simulink model "spacecraft2"  (R2022b)
settings: Solver=ode45  StartTime=0.0  StopTime=tf  RelTol=1e-12  AbsTol=1e-12
values from neighbouring files (symbols this model uses):
  acc = 0.5*pi/180    (= 0.00872664625997)    [runsimulink.m]
  angle0 = [0 0 0]'    [runsimulink.m]
  Jb_cg = diag([90 70 60])    [main.m]    (also in runsimulink.m)
  x0 = [rvi_0;qb_i0;wb_bi0]'    [runsimulink.m]
settings Model: Creator=fg7823  LastModifiedBy=dopestmmac
settings DebuggingCC: UnconnectedInputMsg=warning  UnconnectedOutputMsg=warning  UnconnectedLineMsg=warning
settings ModelReferenceCC: EnableRefExpFcnMdlSchedulingChecks=on
settings RTWCC: DLArmComputeVersion=19.05

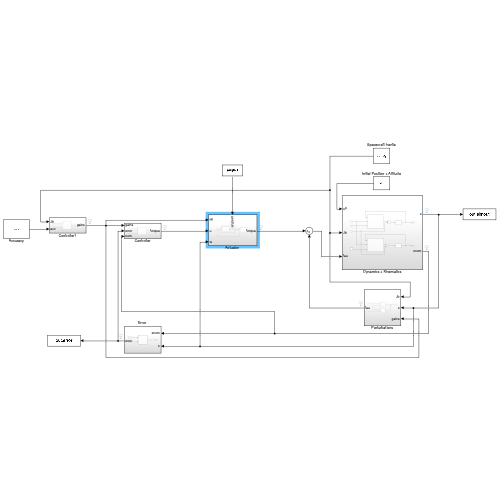
[thumbnail: Simulink's stored preview of the top-level diagram]
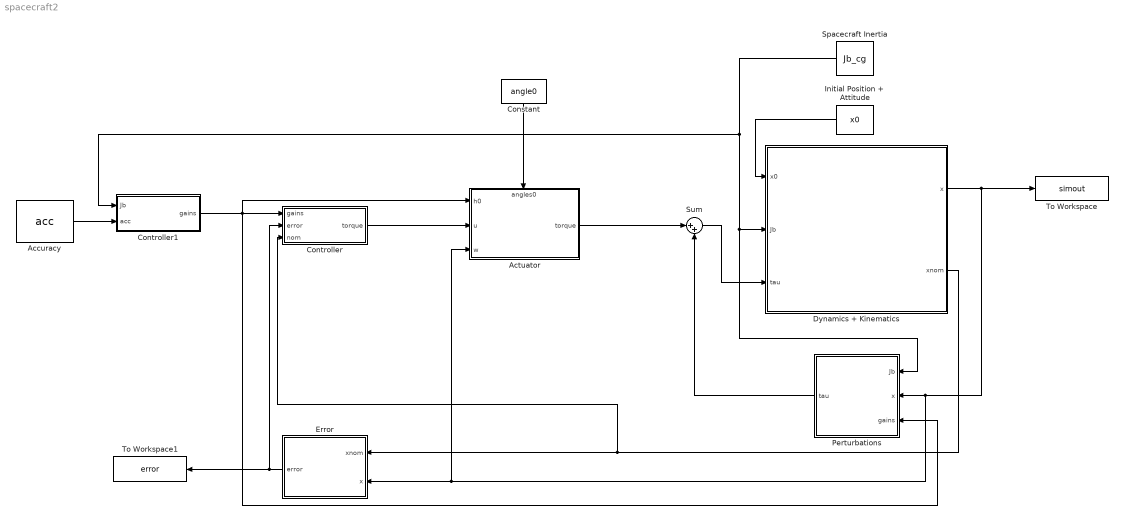
== system spacecraft2 ==
  Accuracy : Constant  Value=acc
  "Actuator " : Subsystem
      settings: PortSchema="{\"entries\":[{\"content\":{\"sides\":[{\"content\":{\"connectorIds\":[\"In1\",\"In2\",\"In3\"]},\"type\":\"ConnectorPlacement.EquallySpacedRectSide\",\"uuid\":\"5f27c84e-cce5-4eac-9877-9210f497f153\"},{\"content\":{\"connectorIds\":[\"Out1\"],\"side\":\"RIGHT\"},\"type\":\"ConnectorPlacement.EquallySpacedRectSide\",\"uuid\":\"a466bbdb-492f-41de-a900-9cb886f81e3e\"},{\"content\":{\"connectorIds\":[\"In4\"],\"side\":\"TOP\"},\"type\":\"ConnectorPlacement.EquallySpacedRectSide\",\"uuid\":\"03fb3c46-a5e4-4bdc-953c-ec3813d7b557\"},{\"content\":{\"connectorIds\":[],\"side\":\"BOTTOM\"},\"type\":\"ConnectorPlacement.EquallySpacedRectSide\",\"uuid\":\"bd57d3c1-5596-4982-b272-865ebb4241ce\"}]},\"type\":\"ConnectorPlacement.EquallySpacedConnector\",\"uuid\":\"40601c32-580e-43fd-8255-02ff6b55ccd6\"}],\"packageUris\":[\"http://schema.mathworks.com/mf0/Connector/R2020b\"],\"version\":\"1.0\"}"
  Constant : Constant  Value=angle0
  Controller : Subsystem
  Controller1 : Subsystem
  Dynamics + Kinematics : Subsystem
  "Error " : Subsystem
  Initial Position + Attitude : Constant  Value=x0
  Perturbations : Subsystem
  Spacecraft Inertia : Constant  Value=Jb_cg
  Sum : Sum  Inputs=|++
  To Workspace : ToWorkspace  VariableName=simout  SampleTime=-1
  To Workspace1 : ToWorkspace  VariableName=error  SampleTime=-1
  wires:
  Spacecraft Inertia/1 -> Controller1/1(Jb), Dynamics + Kinematics/2(Jb), Perturbations/1(Jb)
  Initial Position + Attitude/1 -> Dynamics + Kinematics/1(x0)
  Dynamics + Kinematics/1(x) -> To Workspace/1, Perturbations/2(x), "Actuator "/3(w), "Error "/2(x)
  Dynamics + Kinematics/2(xnom) -> Controller/3(nom), "Error "/1(xnom)
  "Error "/1(error) -> To Workspace1/1, Controller/2(error)
  Sum/1 -> Dynamics + Kinematics/3(tau)
  Controller1/1(gains) -> Controller/1(gains), "Actuator "/1(h0), Perturbations/3(gains)
  Accuracy/1 -> Controller1/2(acc)
  Perturbations/1(tau) -> Sum/2
  Controller/1(torque) -> "Actuator "/2(u)
  Constant/1 -> "Actuator "/4(angles0)
  "Actuator "/1(torque) -> Sum/1

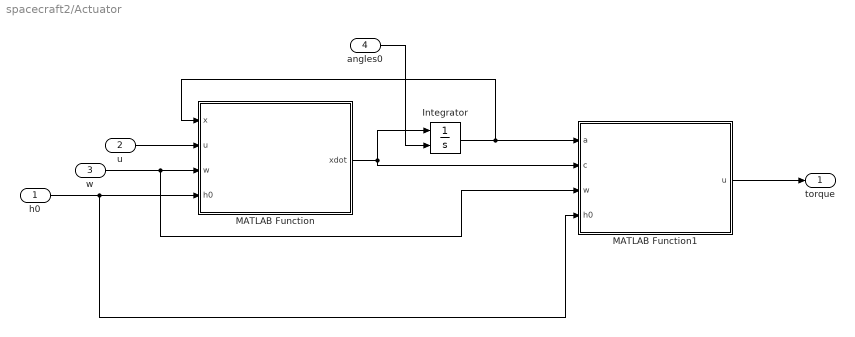
== system spacecraft2/Actuator  ==
  h0 : Inport
  u : Inport  Port=2
  w : Inport  Port=3
  angles0 : Inport  Port=4
  Integrator : Integrator  InitialConditionSource=external
  MATLAB Function : MATLAB Function  TreatAsAtomicUnit=on
  MATLAB Function1 : MATLAB Function  TreatAsAtomicUnit=on
  torque : Outport
  wires:
  MATLAB Function/1(xdot) -> MATLAB Function1/2(c), Integrator/1
  Integrator/1 -> MATLAB Function1/1(a), MATLAB Function/1(x)
  w/1 -> MATLAB Function1/3(w), MATLAB Function/3(w)
  u/1 -> MATLAB Function/2(u)
  angles0/1 -> Integrator/2
  h0/1 -> MATLAB Function1/4(h0), MATLAB Function/4(h0)
  MATLAB Function1/1(u) -> torque/1

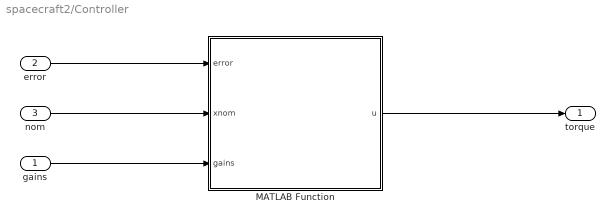
== system spacecraft2/Controller ==
  gains : Inport
  error : Inport  Port=2
  nom : Inport  Port=3
  MATLAB Function : MATLAB Function  TreatAsAtomicUnit=on
  torque : Outport
  wires:
  error/1 -> MATLAB Function/1(error)
  MATLAB Function/1(u) -> torque/1
  nom/1 -> MATLAB Function/2(xnom)
  gains/1 -> MATLAB Function/3(gains)

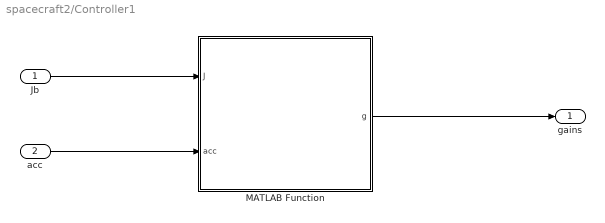
== system spacecraft2/Controller1 ==
  Jb : Inport
  acc : Inport  Port=2
  MATLAB Function : MATLAB Function  TreatAsAtomicUnit=on
  gains : Outport
  wires:
  MATLAB Function/1(g) -> gains/1
  Jb/1 -> MATLAB Function/1(J)
  acc/1 -> MATLAB Function/2(acc)

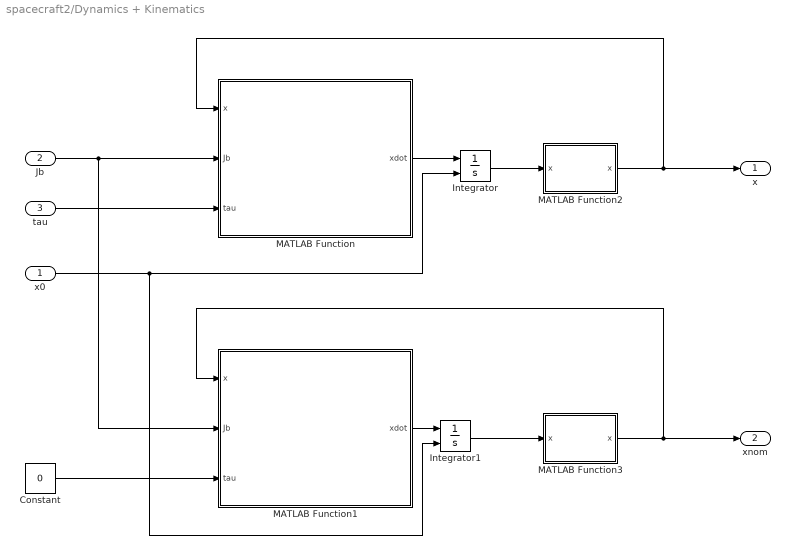
== system spacecraft2/Dynamics + Kinematics ==
  x0 : Inport
  Jb : Inport  Port=2
  tau : Inport  Port=3
  Constant : Constant  Value=0
  Integrator : Integrator  InitialConditionSource=external
  Integrator1 : Integrator  InitialConditionSource=external
  MATLAB Function : MATLAB Function  TreatAsAtomicUnit=on
  MATLAB Function1 : MATLAB Function  TreatAsAtomicUnit=on
  MATLAB Function2 : MATLAB Function  TreatAsAtomicUnit=on
  MATLAB Function3 : MATLAB Function  TreatAsAtomicUnit=on
  x : Outport
  xnom : Outport  Port=2
  wires:
  Jb/1 -> MATLAB Function1/2(Jb), MATLAB Function/2(Jb)
  x0/1 -> Integrator/2, Integrator1/2
  MATLAB Function/1(xdot) -> Integrator/1
  tau/1 -> MATLAB Function/3(tau)
  Integrator/1 -> MATLAB Function2/1("x ")
  MATLAB Function1/1(xdot) -> Integrator1/1
  Integrator1/1 -> MATLAB Function3/1("x ")
  Constant/1 -> MATLAB Function1/3(tau)
  MATLAB Function2/1(x) -> x/1, MATLAB Function/1(x)
  MATLAB Function3/1(x) -> xnom/1, MATLAB Function1/1(x)

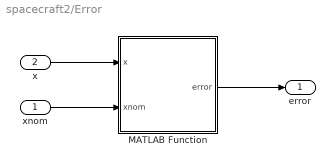
== system spacecraft2/Error  ==
  xnom : Inport
  x : Inport  Port=2
  MATLAB Function : MATLAB Function  TreatAsAtomicUnit=on
  error : Outport
  wires:
  x/1 -> MATLAB Function/1(x)
  xnom/1 -> MATLAB Function/2(xnom)
  MATLAB Function/1(error) -> error/1

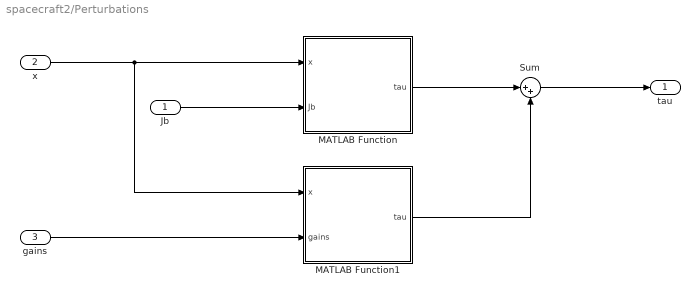
== system spacecraft2/Perturbations ==
  Jb : Inport
  x : Inport  Port=2
  gains : Inport  Port=3
  MATLAB Function : MATLAB Function  TreatAsAtomicUnit=on
  MATLAB Function1 : MATLAB Function  TreatAsAtomicUnit=on
  Sum : Sum  Inputs=|++
  tau : Outport
  wires:
  x/1 -> MATLAB Function1/1(x), MATLAB Function/1(x)
  Jb/1 -> MATLAB Function/2(Jb)
  MATLAB Function/1(tau) -> Sum/1
  MATLAB Function1/1(tau) -> Sum/2
  Sum/1 -> tau/1
  gains/1 -> MATLAB Function1/2(gains)

== matlab function spacecraft2/Perturbations/MATLAB Function ==
  data: x input; tau output; Jb input
function tau = gravitygradient(x,Jb)
    G    = 6.6743e-11;                    % m3/kgs2
    m_e  = 5.97219e+24;
    n    = sqrt(G*m_e/(400e+3 + 6.3781e+6)^3);
    ri   = x(1:3);
    qb_i = x(7:10);
    rb   = Tq(qb_i)*(-ri);
    db   = rb/norm(rb);
    tau  = 3*cross(db,Jb*db)*n^2;
end

== matlab function spacecraft2/Dynamics + Kinematics/MATLAB Function ==
  data: x input; xdot output; Jb input; tau input
function xdot = propagation(x,Jb,tau)
    G           = 6.6743e-11;                    % m3/kgs2
    m_e         = 5.97219e+24;   
    % Unpacking states
    ri          = x(1:3);
    vi          = x(4:6);
    qb_i        = x(7:10);
    wb_bi       = x(11:13);
    xdot        = zeros(13,1);
    % Propagation of position & velocity 
    xdot(1:3)   = vi;
    xdot(4:6)   = -G*m_e*ri/(norm(ri)^3);
    % Propagation of kinematics
    xdot(7:10)  = otimes([wb_bi; 0],qb_i)/2;
    % Propagation of dynamics
    xdot(11:13) = inv(Jb)*(-cross(wb_bi,Jb*wb_bi) + tau);
end

== matlab function spacecraft2/Dynamics + Kinematics/MATLAB Function1 ==
  data: x input; xdot output; Jb input; tau input
function xdot = propagation(x,Jb,tau)
    G           = 6.6743e-11;                    % m3/kgs2
    m_e         = 5.97219e+24;   
    % Unpacking states
    ri          = x(1:3);
    vi          = x(4:6);
    qb_i        = x(7:10);
    wb_bi       = x(11:13);
    xdot        = zeros(13,1);
    % Propagation of position & velocity 
    xdot(1:3)   = vi;
    xdot(4:6)   = -G*m_e*ri/(norm(ri)^3);
    % Propagation of kinematics
    xdot(7:10)  = otimes([wb_bi; 0],qb_i)/2;
    % Propagation of dynamics
    xdot(11:13) = inv(Jb)*(-cross(wb_bi,Jb*wb_bi) + tau);
end

== matlab function spacecraft2/Error /MATLAB Function ==
  data: x input; error output; xnom input
function error = error(x,xnom)
    q    = x(7:10);
    qnom = xnom(7:10);
    w    = x(11:13);
    wnom = xnom(11:13);
    
    qerror = otimes(q,star(qnom));
    werror = w - Tq(qerror)*wnom;
    
    error  = [qerror;werror];
end

== matlab function spacecraft2/Controller/MATLAB Function ==
  data: error input; u output; xnom input; gains input
function u = controller(error,xnom,gains)

    G    = 6.6743e-11;                    % m3/kgs2
    m_e  = 5.97219e+24;
    
    qerror  = error(1:4);
    werror  = error(5:7);
    wnom    = xnom(11:13);
    
    dtheta1 = 2*atan2(qerror(1),qerror(4));
    dtheta2 = 2*atan2(qerror(2),qerror(4));
    dtheta3 = 2*atan2(qerror(3),qerror(4));
    dtheta  = [dtheta1;dtheta2;dtheta3];
    
    dthetadot = werror - cross(wnom,dtheta);
    
    kp1   = gains(1);
    kd1   = gains(2);
    gamma = gains(3);
    kp3   = gains(4);
    kd3   = gains(5);
    h0    = gains(6);
    n     = sqrt(G*m_e/(400e+3 + 6.3781e+6)^3);
    
    u1    = -kp1*dtheta(1) - kd1*dthetadot(1)  + n*h0*dtheta(1);
    u2    = gamma*kp1*dtheta(1) + gamma*kd1*dthetadot(1) - h0*dthetadot(1);
    u3    = -kp3*dtheta(3) - kd3*dthetadot(3);
    
    u = [u1;u2;u3];
end

== matlab function spacecraft2/Controller1/MATLAB Function ==
  data: g output; J input; acc input
function g = gains(J,acc)

    G     = 6.6743e-11;                    % m3/kgs2
    m_e   = 5.97219e+24;
    n     = sqrt(G*m_e/(400e+3 + 6.3781e+6)^3);
    sf    = 2;
    tmax  = 6e-5;
    
    kp3   = sf*(J(3,3)*tmax/acc + 3*(J(2,2)-J(1,1))*n^2);
    kd3   = 2*J(3,3)*sqrt(kp3/J(3,3) - 3*((J(2,2)-J(1,1))/J(3,3))*n^2);
    
    h0    = 2*(3*J(1,1)*n^2)/(acc*n);
    w2n2  = n*h0/J(2,2);
    gamma = 2*J(2,2)*sqrt(w2n2)/h0;
    
    kp1   = sf*(sqrt(J(1,1))*gamma*h0/(2*J(2,2)))^2;
    kd1   = 2*sqrt(J(1,1)/kp1)*kp1;
    
    g     = [kp1 kd1 gamma kp3 kd3 h0]';
end

== matlab function spacecraft2/Dynamics + Kinematics/MATLAB Function2 ==
  data: x input; x output
function x = normalize(x)
     x(7:10) = x(7:10)/norm(x(7:10));
end

== matlab function spacecraft2/Dynamics + Kinematics/MATLAB Function3 ==
  data: x input; x output
function x = normalize(x)
     x(7:10) = x(7:10)/norm(x(7:10));
end

== matlab function spacecraft2/Perturbations/MATLAB Function1 ==
  data: x input; tau output; gains input
function tau = momentumwheel(x,gains)
    wb_bi = x(11:13);
    tau  = -cross(wb_bi,[0 0 gains(end)]');
end

== matlab function spacecraft2/Actuator /MATLAB Function ==
  data: x input; u input; xdot output; w input; h0 input
function xdot = actuatorprop(x,u,w,h0)

    h0      = h0(end);
    w       = w(11:13);
    alphah0 = x(1);
    delh0   = x(2);
    betah0  = x(3);

    xdot  = -u - cross(w,[alphah0 h0 + delh0 betah0]'); 
end

== matlab function spacecraft2/Actuator /MATLAB Function1 ==
  data: a input; c input; u output; w input; h0 input
function u = actuatortorque(a,c,w,h0)

    h0      = h0(end);
    w       = w(11:13);
    a(2)    = a(2) + h0;
    u       = -c - cross(w,a);
end
